simulink model "Data_process"  (R2020b)
settings: Solver=FixedStepDiscrete  StartTime=0.0  StopTime=300  FixedStep=0.04  RelTol=1e-3
InitFcn:
  | %load TRNDataBusPILS.mat
  | %addpath(genpath(cd))
  | 
  | % Add DataBus Path
  | addpath(',,/');
  | addpath('../MAP/');
  | addpath('../MAP/MAP_DB');
  | addpath('../MAP/DVOF');
  | addpath(genpath(cd));
  | load('BusStructureTRN.mat');
libraries: aerolibconvert2 x14, simulink_extras x2
settings Model: Creator=Seungjo Oh  LastModifiedBy=ASCL
settings DataIOCC: ReturnWorkspaceOutputs=off
settings OptimizationCC: DefaultParameterBehavior=Inlined  UseDivisionForNetSlopeComputation=on  GainParamInheritBuiltInType=on  UseFloatMulNetSlope=on  InlineInvariantSignals=on  PassReuseOutputArgsAs=Individual arguments  ZeroExternalMemoryAtStartup=off  ZeroInternalMemoryAtStartup=off  NoFixptDivByZeroProtection=on  EfficientFloat2IntCast=on  LifeSpan=1  OptimizeBlockOrder=speed  DifferentSizesBufferReuse=on  EfficientTunableParamExpr=on
settings DebuggingCC: ParameterTunabilityLossMsg=error  ArithmeticOperatorsInVariantConditions=warning
settings HardwareCC: ProdBitPerPointer=32  ProdBitPerSizeT=32  ProdBitPerPtrDiffT=32  ProdLargestAtomicInteger=Long  ProdLargestAtomicFloat=Double  ProdEndianess=BigEndian  ProdWordSize=32  ProdLongLongMode=on  ProdHWDeviceType=Freescale->MPC83xx  TargetBitPerPointer=64  TargetBitPerSizeT=64  TargetBitPerPtrDiffT=64  TargetLongLongMode=on  TargetIntDivRoundTo=Zero  TargetEndianess=LittleEndian  TargetWordSize=64  TargetHWDeviceType=MATLAB Host
settings SFSimCC: SimUseLocalCustomCode=off  SimParseCustomCode=off  MATLABDynamicMemAlloc=off  CustomCodeUndefinedFunction=UseInterfaceOnly
settings SFSimCC: SimCustomHeaderCode=|
  | #include "MAP.h"
  | #include "MAPDATA.h"
  | #include "DVOF.h"
  | #include "userDefined.h"
settings SFSimCC: SimUserSources=|
  | MAP.c
  | DVOF.c
  | userDefined.c
settings SFSimCC: SimUserLibraries=|
  | WS2_32.LIB
  | MAPd.LIB
settings RTWCC: Description=Embedded Coder  SystemTargetFile=ert.tlc  TemplateMakefile=ert_default_tmf  GenerateReport=on  RTWUseLocalCustomCode=off  RTWUseSimCustomCode=on  LaunchReport=on
settings RTWCC: CustomHeaderCode=|
  | #include "MAP.h"
  | #include "MAPDATA.h"
  | #include "DVOF.h"
  | #include "userDefined.h"
settings RTWCC: CustomSource=|
  | MAP.c
  | DVOF.c
  | userDefined.c
settings RTWCC: CustomLibrary=|
  | WS2_32.LIB
  | MAPd.LIB
settings CodeAppCC: ForceParamTrailComments=on  IgnoreCustomStorageClasses=off  OperatorAnnotations=on  SimulinkDataObjDesc=on  SFDataObjDesc=on  InsertBlockDesc=on
settings ERTTargetCC: TargetLangStandard=C99 (ISO)  GenerateSampleERTMain=on  IncludeMdlTerminateFcn=off  CombineSignalStateStructs=on  SupportAbsoluteTime=off  SupportComplex=off  InlinedParameterPlacement=NonHierarchical  ERTCustomFileTemplate=example_file_process.tlc  ERTFilePackagingFormat=CompactWithDataFile

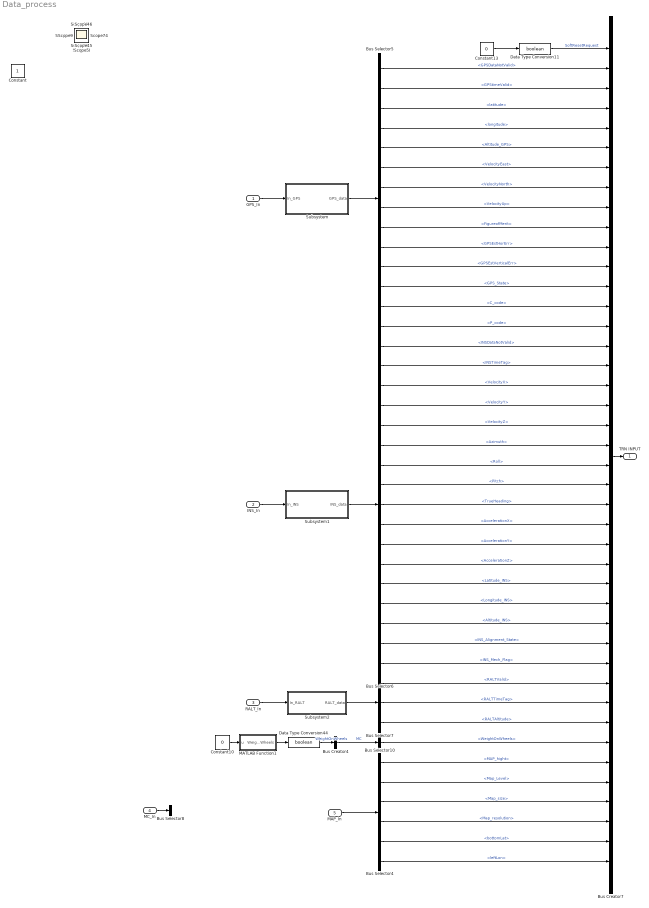
== system Data_process ==
  GPS_In : Inport  OutDataTypeStr=Bus: BUS_SENSOR_GPS  BusOutputAsStruct=on
  INS_In : Inport  Port=2  OutDataTypeStr=Bus: BUS_SENSOR_INS  BusOutputAsStruct=on
  RALT_In : Inport  Port=3  OutDataTypeStr=Bus: BUS_SENSOR_RALT  BusOutputAsStruct=on
  MC_In : Inport  Port=4  OutDataTypeStr=Bus: TRN_MC  BusOutputAsStruct=on
  MAP_In : Inport  Port=5  OutDataTypeStr=Bus: TRN_MAP  BusOutputAsStruct=on
  Bus Creator4 : BusCreator  Inputs=1  OutDataTypeStr=Bus: TRN_MC
  Bus Creator7 : BusCreator  Inputs=42  OutDataTypeStr=Bus: TRNInput
  Bus Selector10 : BusSelector  OutputSignals=WeightOnWheels
  Bus Selector4 : BusSelector  OutputSignals=MAP_hight,Map_Level,Map_size,Map_resolution,bottomLat,leftLon
  Bus Selector5 : BusSelector  OutputSignals=GPSDataNotValid,GPStimeValid,latitude,longitude,Altitude_GPS,VelocityEast,VelocityNorth,VelocityUp,FigureofMerit,GPSEstHorErr,GPSEstVerticalErr,GPS_State,C_code,P_code
  Bus Selector6 : BusSelector  OutputSignals=INSDataNotValid,INSTimeTag,VelocityX,VelocityY,VelocityZ,Azimuth,Roll,Pitch,TrueHeading,AccelerationX,AccelerationY,AccelerationZ,Latitude_INS,Longitude_INS,Altitude_INS,INS_Alignment_State,INS_Mech_Flag
  Bus Selector7 : BusSelector  OutputSignals=RALTValid,RALTTimeTag,RALTAltitude
  Bus Selector8 : BusSelector  OutputSignals=WeightOnWheels
  Constant10 : Constant  Value=0
  Constant13 : Constant  Value=0
  Data Type Conversion11 : DataTypeConversion  OutDataTypeStr=boolean
  Data Type Conversion44 : DataTypeConversion  OutDataTypeStr=boolean
  MATLAB Function1 : MATLAB Function  TreatAsAtomicUnit=on
  Subsystem : Subsystem
  Subsystem1 : Subsystem
  Subsystem2 : Subsystem
  TRN INPUT : Outport  OutDataTypeStr=Bus: TRNInput  VectorParamsAs1DForOutWhenUnconnected=off  BusOutputAsStruct=on
  Constant : Constant  IOType=siggen
  Scope{,2,4..5,7,9,11..22,29..30,34..36,40..46} (30 alike) : Scope
  wires:
  Bus Selector5/1 -> Bus Creator7/2  "<GPSDataNotValid>"
  Bus Selector5/6 -> Bus Creator7/7  "<VelocityEast>"
  Bus Selector5/11 -> Bus Creator7/12  "<GPSEstVerticalErr>"
  Bus Selector5/9 -> Bus Creator7/10  "<FigureofMerit>"
  Bus Selector5/10 -> Bus Creator7/11  "<GPSEstHorErr>"
  Bus Selector5/7 -> Bus Creator7/8  "<VelocityNorth>"
  Bus Selector5/4 -> Bus Creator7/5  "<longitude>"
  Bus Selector5/2 -> Bus Creator7/3  "<GPStimeValid>"
  Bus Selector5/3 -> Bus Creator7/4  "<latitude>"
  Bus Selector5/8 -> Bus Creator7/9  "<VelocityUp>"
  Bus Selector5/5 -> Bus Creator7/6  "<Altitude_GPS>"
  Bus Selector5/12 -> Bus Creator7/13  "<GPS_State>"
  Bus Selector5/13 -> Bus Creator7/14  "<C_code>"
  Bus Selector5/14 -> Bus Creator7/15  "<P_code>"
  Bus Selector6/1 -> Bus Creator7/16  "<INSDataNotValid>"
  Bus Selector6/2 -> Bus Creator7/17  "<INSTimeTag>"
  Bus Selector6/3 -> Bus Creator7/18  "<VelocityX>"
  Bus Selector6/4 -> Bus Creator7/19  "<VelocityY>"
  Bus Selector6/5 -> Bus Creator7/20  "<VelocityZ>"
  Bus Selector6/6 -> Bus Creator7/21  "<Azimuth>"
  Bus Selector6/7 -> Bus Creator7/22  "<Roll>"
  Bus Selector6/8 -> Bus Creator7/23  "<Pitch>"
  Bus Selector6/9 -> Bus Creator7/24  "<TrueHeading>"
  Bus Selector6/10 -> Bus Creator7/25  "<AccelerationX>"
  Bus Selector6/11 -> Bus Creator7/26  "<AccelerationY>"
  Bus Selector6/12 -> Bus Creator7/27  "<AccelerationZ>"
  MC_In/1 -> Bus Selector8/1
  Constant10/1 -> MATLAB Function1/1(u)
  Bus Selector6/14 -> Bus Creator7/29  "<Longitude_INS>"
  Bus Selector6/15 -> Bus Creator7/30  "<Altitude_INS>"
  Bus Selector6/16 -> Bus Creator7/31  "<INS_Alignment_State>"
  Bus Selector6/17 -> Bus Creator7/32  "<INS_Mech_Flag>"
  Bus Creator4/1 -> Bus Selector10/1  "MC"
  Bus Selector7/1 -> Bus Creator7/33  "<RALTValid>"
  Bus Selector7/2 -> Bus Creator7/34  "<RALTTimeTag>"
  Bus Selector7/3 -> Bus Creator7/35  "<RALTAltitude>"
  Bus Selector4/2 -> Bus Creator7/38  "<Map_Level>"
  Bus Selector4/3 -> Bus Creator7/39  "<Map_size>"
  Bus Selector4/4 -> Bus Creator7/40  "<Map_resolution>"
  Bus Selector4/5 -> Bus Creator7/41  "<bottomLat>"
  Bus Selector4/6 -> Bus Creator7/42  "<leftLon>"
  MATLAB Function1/1(WeightOnWheels) -> Data Type Conversion44/1
  Data Type Conversion44/1 -> Bus Creator4/1  "WeightOnWheels"
  Bus Selector6/13 -> Bus Creator7/28  "<Latitude_INS>"
  Bus Selector10/1 -> Bus Creator7/36  "<WeightOnWheels>"
  Bus Selector4/1 -> Bus Creator7/37  "<MAP_hight>"
  Bus Creator7/1 -> TRN INPUT/1
  MAP_In/1 -> Bus Selector4/1
  Constant13/1 -> Data Type Conversion11/1
  Data Type Conversion11/1 -> Bus Creator7/1  "SoftResetRequest"
  GPS_In/1 -> Subsystem/1(In_GPS)
  Subsystem/1(GPS_data) -> Bus Selector5/1
  INS_In/1 -> Subsystem1/1(In_INS)
  Subsystem1/1(INS_data) -> Bus Selector6/1
  RALT_In/1 -> Subsystem2/1(In_RALT)
  Subsystem2/1(RALT_data) -> Bus Selector7/1

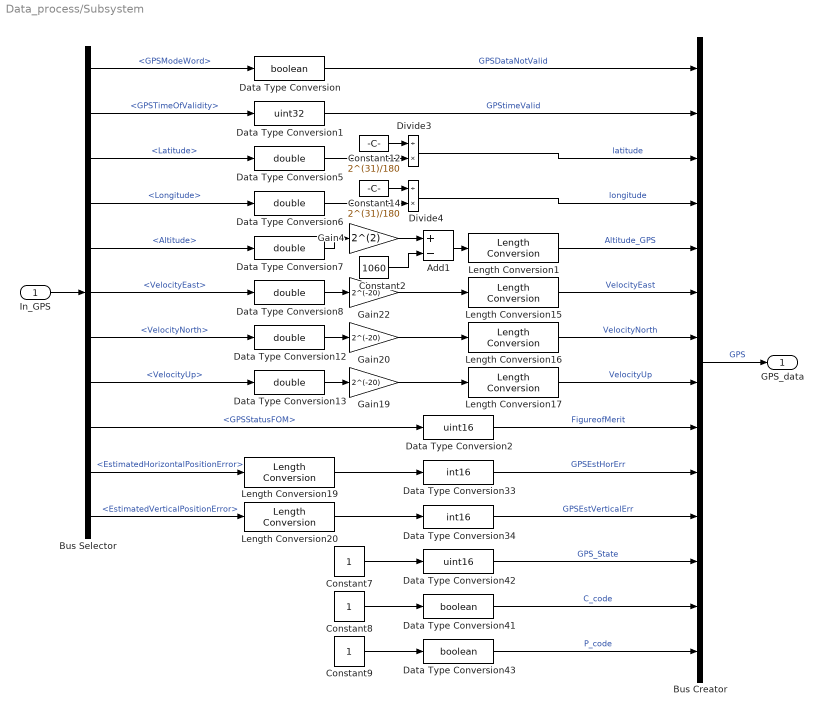
== system Data_process/Subsystem ==
  In_GPS : Inport
  Add1 : Sum  Inputs=+-
  Bus Creator : BusCreator  Inputs=14  OutDataTypeStr=Bus: TRN_GPS
  Bus Selector : BusSelector  OutputSignals=GPSModeWord,GPSTimeOfValidity,Latitude,Longitude,Altitude,VelocityEast,VelocityNorth,VelocityUp,GPSStatusFOM,EstimatedHorizontalPositionError,EstimatedVerticalPositionError
  Constant12 : Constant  Value=2^(31)/180
  Constant14 : Constant  Value=2^(31)/180
  Constant2 : Constant  Value=1060
  Constant7 : Constant
  Constant8 : Constant
  Constant9 : Constant
  Data Type Conversion : DataTypeConversion  OutDataTypeStr=boolean
  Data Type Conversion1 : DataTypeConversion  OutDataTypeStr=uint32
  Data Type Conversion{5..8,12..13} (6 alike) : DataTypeConversion  OutDataTypeStr=double
  Data Type Conversion2 : DataTypeConversion  OutDataTypeStr=uint16
  Data Type Conversion33 : DataTypeConversion  OutDataTypeStr=int16
  Data Type Conversion34 : DataTypeConversion  OutDataTypeStr=int16
  Data Type Conversion41 : DataTypeConversion  OutDataTypeStr=boolean
  Data Type Conversion42 : DataTypeConversion  OutDataTypeStr=uint16
  Data Type Conversion43 : DataTypeConversion  OutDataTypeStr=boolean
  Divide3 : Product  Inputs=/*
  Divide4 : Product  Inputs=/*
  Gain19 : Gain  Gain=2^(-20)
  Gain20 : Gain  Gain=2^(-20)
  Gain22 : Gain  Gain=2^(-20)
  Gain4 : Gain  Gain=2^(2)
  Length Conversion{1,15..17,19..20} (6 alike) : aerolibconvert2/Length Conversion  IU=ft  OU=m
  GPS_data : Outport
  wires:
  Length Conversion1/1 -> Bus Creator/5  "Altitude_GPS"
  Bus Selector/1 -> Data Type Conversion/1  "<GPSModeWord>"
  Bus Selector/7 -> Data Type Conversion12/1  "<VelocityNorth>"
  Bus Selector/2 -> Data Type Conversion1/1  "<GPSTimeOfValidity>"
  Bus Selector/3 -> Data Type Conversion5/1  "<Latitude>"
  Gain4/1 -> Add1/1
  Data Type Conversion33/1 -> Bus Creator/10  "GPSEstHorErr"
  Bus Selector/5 -> Data Type Conversion7/1  "<Altitude>"
  Data Type Conversion8/1 -> Gain22/1
  Data Type Conversion41/1 -> Bus Creator/13  "C_code"
  Bus Selector/11 -> Length Conversion20/1  "<EstimatedVerticalPositionError>"
  Gain20/1 -> Length Conversion16/1
  Bus Selector/10 -> Length Conversion19/1  "<EstimatedHorizontalPositionError>"
  Divide3/1 -> Bus Creator/3  "latitude"
  Bus Selector/6 -> Data Type Conversion8/1  "<VelocityEast>"
  Data Type Conversion13/1 -> Gain19/1
  Data Type Conversion6/1 -> Divide4/2
  Data Type Conversion34/1 -> Bus Creator/11  "GPSEstVerticalErr"
  Data Type Conversion42/1 -> Bus Creator/12  "GPS_State"
  Gain22/1 -> Length Conversion15/1
  Length Conversion20/1 -> Data Type Conversion34/1
  Data Type Conversion5/1 -> Divide3/2
  Add1/1 -> Length Conversion1/1
  Data Type Conversion1/1 -> Bus Creator/2  "GPStimeValid"
  Gain19/1 -> Length Conversion17/1
  Constant8/1 -> Data Type Conversion41/1
  Data Type Conversion2/1 -> Bus Creator/9  "FigureofMerit"
  Data Type Conversion7/1 -> Gain4/1
  Bus Selector/8 -> Data Type Conversion13/1  "<VelocityUp>"
  Constant7/1 -> Data Type Conversion42/1
  Data Type Conversion/1 -> Bus Creator/1  "GPSDataNotValid"
  Bus Selector/4 -> Data Type Conversion6/1  "<Longitude>"
  Bus Selector/9 -> Data Type Conversion2/1  "<GPSStatusFOM>"
  Length Conversion17/1 -> Bus Creator/8  "VelocityUp"
  Length Conversion16/1 -> Bus Creator/7  "VelocityNorth"
  Bus Creator/1 -> GPS_data/1  "GPS"
  Data Type Conversion12/1 -> Gain20/1
  Constant2/1 -> Add1/2
  Length Conversion15/1 -> Bus Creator/6  "VelocityEast"
  Length Conversion19/1 -> Data Type Conversion33/1
  Divide4/1 -> Bus Creator/4  "longitude"
  Constant9/1 -> Data Type Conversion43/1
  In_GPS/1 -> Bus Selector/1
  Constant14/1 -> Divide4/1
  Constant12/1 -> Divide3/1
  Data Type Conversion43/1 -> Bus Creator/14  "P_code"

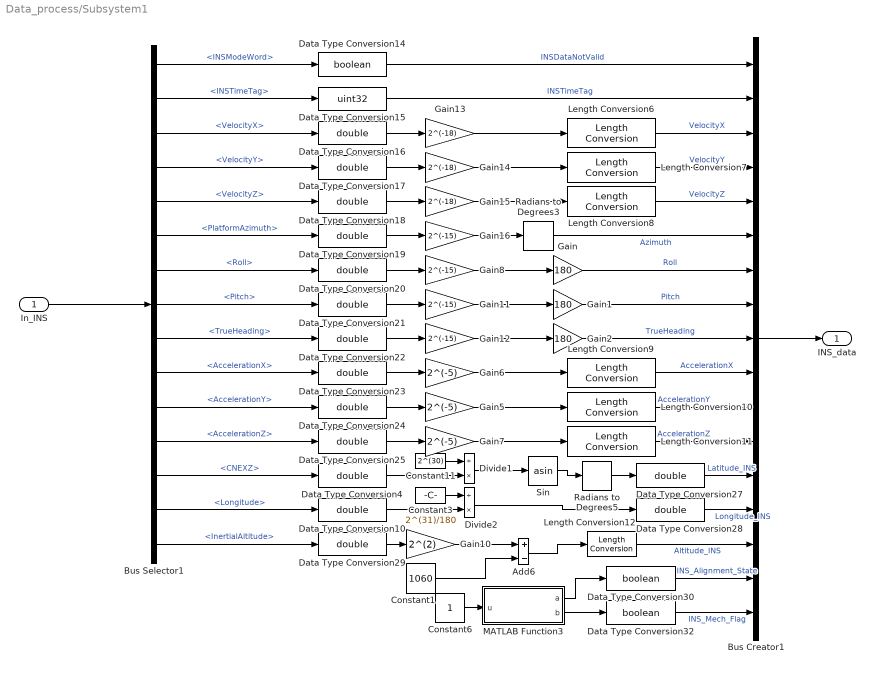
== system Data_process/Subsystem1 ==
  In_INS : Inport
  Add6 : Sum  Inputs=+-
  Bus Creator1 : BusCreator  Inputs=17  OutDataTypeStr=Bus: TRN_INS
  Bus Selector1 : BusSelector  OutputSignals=INSModeWord,INSTimeTag,VelocityX,VelocityY,VelocityZ,PlatformAzimuth,Roll,Pitch,TrueHeading,AccelerationX,AccelerationY,AccelerationZ,CNEXZ,Longitude,InertialAltitude
  Constant1 : Constant  Value=1060
  Constant11 : Constant  Value=2^(30)
  Constant3 : Constant  Value=2^(31)/180
  Constant6 : Constant
  Data Type Conversion{4,10,16..25,27..29} (15 alike) : DataTypeConversion  OutDataTypeStr=double
  Data Type Conversion14 : DataTypeConversion  OutDataTypeStr=boolean
  Data Type Conversion15 : DataTypeConversion  OutDataTypeStr=uint32
  Data Type Conversion30 : DataTypeConversion  OutDataTypeStr=boolean
  Data Type Conversion32 : DataTypeConversion  OutDataTypeStr=boolean
  Divide1 : Product  Inputs=/*
  Divide2 : Product  Inputs=/*
  Gain : Gain  Gain=180
  Gain1 : Gain  Gain=180
  Gain10 : Gain  Gain=2^(2)
  Gain{8,11..12,16} (4 alike) : Gain  Gain=2^(-15)
  Gain13 : Gain  Gain=2^(-18)
  Gain14 : Gain  Gain=2^(-18)
  Gain15 : Gain  Gain=2^(-18)
  Gain2 : Gain  Gain=180
  Gain5 : Gain  Gain=2^(-5)
  Gain6 : Gain  Gain=2^(-5)
  Gain7 : Gain  Gain=2^(-5)
  Length Conversion{6..12} (7 alike) : aerolibconvert2/Length Conversion  IU=ft  OU=m
  MATLAB Function3 : MATLAB Function  TreatAsAtomicUnit=on
  Radians to Degrees3 : simulink_extras/Transformations/Radians to Degrees
  Radians to Degrees5 : simulink_extras/Transformations/Radians to Degrees
  Sin : Trigonometry  Operator=asin
  INS_data : Outport
  wires:
  Length Conversion6/1 -> Bus Creator1/3  "VelocityX"
  Constant6/1 -> MATLAB Function3/1(u)
  MATLAB Function3/2(b) -> Data Type Conversion32/1
  Data Type Conversion32/1 -> Bus Creator1/17  "INS_Mech_Flag"
  Data Type Conversion22/1 -> Gain12/1
  Length Conversion9/1 -> Bus Creator1/10  "AccelerationX"
  Data Type Conversion29/1 -> Gain10/1
  Gain2/1 -> Bus Creator1/9  "TrueHeading"
  Data Type Conversion16/1 -> Gain13/1
  Data Type Conversion28/1 -> Bus Creator1/14  "Longitude_INS"
  Data Type Conversion18/1 -> Gain15/1
  Data Type Conversion15/1 -> Bus Creator1/2  "INSTimeTag"
  Bus Selector1/14 -> Data Type Conversion10/1  "<Longitude>"
  Radians to Degrees5/1 -> Data Type Conversion27/1
  Data Type Conversion24/1 -> Gain5/1
  Sin/1 -> Radians to Degrees5/1
  Constant1/1 -> Add6/2
  Data Type Conversion14/1 -> Bus Creator1/1  "INSDataNotValid"
  Bus Selector1/5 -> Data Type Conversion18/1  "<VelocityZ>"
  Data Type Conversion25/1 -> Gain7/1
  Divide2/1 -> Data Type Conversion28/1
  MATLAB Function3/1(a) -> Data Type Conversion30/1
  Data Type Conversion19/1 -> Gain16/1
  Bus Selector1/10 -> Data Type Conversion23/1  "<AccelerationX>"
  Data Type Conversion20/1 -> Gain8/1
  Bus Selector1/6 -> Data Type Conversion19/1  "<PlatformAzimuth>"
  Data Type Conversion27/1 -> Bus Creator1/13  "Latitude_INS"
  Data Type Conversion23/1 -> Gain6/1
  Bus Selector1/7 -> Data Type Conversion20/1  "<Roll>"
  Bus Selector1/2 -> Data Type Conversion15/1  "<INSTimeTag>"
  Gain11/1 -> Gain1/1
  Bus Selector1/1 -> Data Type Conversion14/1  "<INSModeWord>"
  Bus Selector1/4 -> Data Type Conversion17/1  "<VelocityY>"
  Bus Selector1/3 -> Data Type Conversion16/1  "<VelocityX>"
  Add6/1 -> Length Conversion12/1
  Bus Selector1/15 -> Data Type Conversion29/1  "<InertialAltitude>"
  Bus Selector1/12 -> Data Type Conversion25/1  "<AccelerationZ>"
  Bus Selector1/13 -> Data Type Conversion4/1  "<CNEXZ>"
  Data Type Conversion4/1 -> Divide1/2
  Bus Selector1/9 -> Data Type Conversion22/1  "<TrueHeading>"
  Bus Selector1/11 -> Data Type Conversion24/1  "<AccelerationY>"
  Length Conversion12/1 -> Bus Creator1/15  "Altitude_INS"
  Data Type Conversion21/1 -> Gain11/1
  Length Conversion8/1 -> Bus Creator1/5  "VelocityZ"
  Data Type Conversion17/1 -> Gain14/1
  Gain1/1 -> Bus Creator1/8  "Pitch"
  Length Conversion7/1 -> Bus Creator1/4  "VelocityY"
  Constant3/1 -> Divide2/1
  Length Conversion10/1 -> Bus Creator1/11  "AccelerationY"
  Gain8/1 -> Gain/1
  Gain/1 -> Bus Creator1/7  "Roll"
  Divide1/1 -> Sin/1
  Bus Selector1/8 -> Data Type Conversion21/1  "<Pitch>"
  Data Type Conversion10/1 -> Divide2/2
  Data Type Conversion30/1 -> Bus Creator1/16  "INS_Alignment_State"
  Gain10/1 -> Add6/1
  Radians to Degrees3/1 -> Bus Creator1/6  "Azimuth"
  Length Conversion11/1 -> Bus Creator1/12  "AccelerationZ"
  Constant11/1 -> Divide1/1
  Gain12/1 -> Gain2/1
  Gain16/1 -> Radians to Degrees3/1
  Bus Creator1/1 -> INS_data/1
  In_INS/1 -> Bus Selector1/1
  Gain13/1 -> Length Conversion6/1
  Gain15/1 -> Length Conversion8/1
  Gain14/1 -> Length Conversion7/1
  Gain6/1 -> Length Conversion9/1
  Gain7/1 -> Length Conversion11/1
  Gain5/1 -> Length Conversion10/1

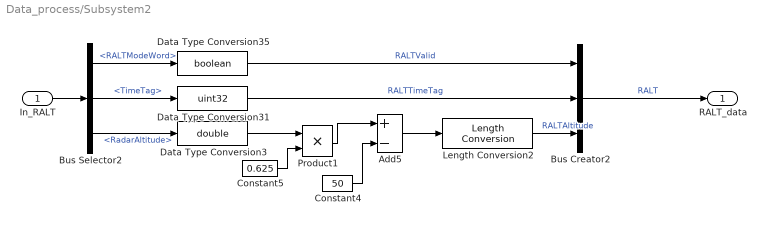
== system Data_process/Subsystem2 ==
  In_RALT : Inport
  Add5 : Sum  Inputs=+-
  Bus Creator2 : BusCreator  Inputs=3  OutDataTypeStr=Bus: TRN_RALT
  Bus Selector2 : BusSelector  OutputSignals=RALTModeWord,TimeTag,RadarAltitude
  Constant4 : Constant  Value=50
  Constant5 : Constant  Value=0.625
  Data Type Conversion3 : DataTypeConversion  OutDataTypeStr=double
  Data Type Conversion31 : DataTypeConversion  OutDataTypeStr=uint32
  Data Type Conversion35 : DataTypeConversion  OutDataTypeStr=boolean
  Length Conversion2 : aerolibconvert2/Length Conversion  IU=ft  OU=m
  Product1 : Product
  RALT_data : Outport
  wires:
  Length Conversion2/1 -> Bus Creator2/3  "RALTAltitude"
  Bus Selector2/1 -> Data Type Conversion35/1  "<RALTModeWord>"
  Bus Selector2/2 -> Data Type Conversion31/1  "<TimeTag>"
  Data Type Conversion31/1 -> Bus Creator2/2  "RALTTimeTag"
  Constant5/1 -> Product1/2
  Product1/1 -> Add5/1
  Data Type Conversion3/1 -> Product1/1
  Bus Selector2/3 -> Data Type Conversion3/1  "<RadarAltitude>"
  Add5/1 -> Length Conversion2/1
  Data Type Conversion35/1 -> Bus Creator2/1  "RALTValid"
  In_RALT/1 -> Bus Selector2/1
  Bus Creator2/1 -> RALT_data/1  "RALT"
  Constant4/1 -> Add5/2

== matlab function Data_process/MATLAB Function1 ==
  data: u input; WeightOnWheels output
function WeightOnWheels  = fcn(u)

% WeightOnWheels
if(u==1)
    WeightOnWheels = true;
else
    WeightOnWheels = false;
end

end

== matlab function Data_process/Subsystem1/MATLAB Function3 ==
  data: u input; a output; b output
function [a,b]  = fcn(u)

% WeightOnWheels
if(u==1)
    a = true;
    b = true;
else
    a = false;
    b = false;
end

end
